simulink library "powerlib_extras"  (Simulink 6.0)
settings: Solver=ode45  SolverMode=SingleTasking  StartTime=0.0  StopTime=10.0  RelTol=1e-3
undefined symbols (not defined in the file or in its folder): Ac, Bc, Cc, Dc, Delay_discrete, dend, DiscIntNeverNeededParam, extra_sc, j, numd, test_alpha, Ts
libraries: powerlib2 x112, powerlib_extras x70, simulink_extras x25, simulink x12, powerlib_models x8
(part 3 of 9)

== system powerlib_extras/Measurements ==
  note: ____ Single-Phase Measurements _____________________________
  note: ____ Three-Phase Measurements _____________________________
  note: ____ Power Measurements __________________________________
  3-Phase Sequence Analyzer : Subsystem  mask(3-Phase Sequence analyzer){f1=60, n=1, seq=Positive}
      mask prompts: f1 "Fundamental frequency f1 (Hz):"; n "Harmonic n (0=DC; 1=fundamental) :"; seq "Sequence :"
      mask help:
      | This block outputs the positive-,  negative- or zero- or all sequence component(s) (Magnitude and Phase)  of a set of three balanced or unbalanced signals  which may contain harmonics. The three sequence components arecomputed as folllows:
      |
      | V1 = 1/3 * (Va + a*Vb  + a^2 *Vc )
      | V2 = 1/3 * (Va + a ^2*Vb  +  a *Vc )
      | V0 = 1/3 * (Va +  Vb  +  Vc )
      | where: Va, Vb, Vc = input phasors at specified frequency
      |            a =exp(j *2pi/3) = 1 < + 120 deg.  complex operator
      |
      | The input contains the vectorized signal of the three [Va Vb Vc] sinusoidal signals
      | Output one and two give respectively the magnitude (peak value) and phase (degrees) of the specified sequence component (s).
      |
      | You can modify any parameter during the simulation in order to obtain the different sequence and  harmonic components of the input. signals.
      |
      | Press Help for more information.
      mask init:
      | Pha20_On=0;
      | k=2-(n==0);
      | a=exp(j*2*pi/3);
      | a2=exp(-j*2*pi/3);
      | switch seq
      | case 1,  % Pos. seq.
      |      PosOn=1;NegOn=0;ZeroOn=0;SelectElement=1;
      | case 2,  % Neg. seq.
      |      PosOn=0;NegOn=1;ZeroOn=0;SelectElement=2;
      | case 3,  % Zero. seq.
      |      PosOn=0;NegOn=0;ZeroOn=1;SelectElement=3;
      | case 4,  % All sequences
      |      PosOn=1;NegOn=1;ZeroOn=1;SelectElement=[1,2,3];Pha20_On=1;
      | end
      mask Help: web(psbhelp)
      mask StyleString: edit,edit,popup(Positive|Negative|Zero|Positive Negative Zero)
  3-phase  Instantaneous  Active & Reactive Power : Subsystem  mask(3-phase instantaneous active and reactive power){}
      mask help:
      | This block computes the 3-phase instantaneous active (P) and reactive (Q) power associated with a periodic set of 3-phase voltages and currents.
      | Note: Result for the instantaneous reactive power (Q) is accurate only for balanced and harmonic-free 3-phase quantities (voltages and currents).
      |
      | Input 1: Vectorized 3-phase  instantaneous voltage (Vabc)
      | Input 2: Vectorized 3-phase instantaneous current (Iabc)
      | Output : Computed PQ vector [P(W) Q(var)]. Current flowing into an RL circuit will produce  positive active and reactive power.
  Active & Reactive Power : Subsystem  mask(Active & Reactive Power ){f1=60}
      mask prompts: f1 "Fundamental frequency (Hz):"
      mask help:
      | This block measures the active power P and reactive power Q  associated with a periodic  set of voltage and current which may contain harmonics. P and Q are calculated by averaging the V.I product with a running window over one cycle of the fundamental frequency so that the powers are evaluated at fundamental frequency.
      |
      | Sign convention: Current flowing into an RL branch will produce positive active and reactive powers.
      mask Help: web(psbhelp)
  Fourier : Subsystem  mask(Fourier analyser){f1=60, n=1}
      mask prompts: f1 "Fundamental frequency f1 (Hz):"; n "Harmonic n (0=DC; 1=fundamental; 2=2nd harm;  ...) :"
      mask help: The Fourier block performs a Fourier analysis of the input signal over a running window of one cycle of the fundamental frequency. First and second outputs return respectively the magnitude and phase (degrees) of the harmonic component specified.
      mask init:
      | k=2-(n==0);
      mask Help: web(psbhelp)
  Mean Value : Subsystem  mask(Mean value){Period=1/60}
      mask prompts: Period "Averaging period (s):"
      mask help: This block uses the running window averaging technique to compute the mean value of the input signal over the specified period.
  Mean Value (linear) : Subsystem  mask(Mean Value (linear)){Freq=60, n=3, Vinit=1}
      mask prompts: Freq "Fundamental frequency (Hz)"; n "Pade order (for linearization)"; Vinit "Initial input:"
      mask help:
      | This block computes the mean value of the input signal over one cycle of the specified fundamental frequency.
      | Pade approximation is used to linearize the one-cycle delay required to compute the mean value.
      mask init:
      | % Pade Approximation:
      | % The coefficients of the Pade approximation are given by the 
      | % recursion   h[k+1] = (N-k)/(2*N-k)/(k+1) * h[k],  h[0] = 1
      | % and 
      | %     exp(-T*s) == Sum { h[k] (-T*s)^k } / Sum { h[k] (T*s)^k }
      | %
      | T=1/Freq;
      | a = zeros(1,n+1);   a(1) = 1;
      | b = zeros(1,n+1);   b(1) = 1;
      | for k = 1:n,
      | 	fact = T*(n-k+1)/(2*n-k+1)/k;
      | 	a(k+1) = (-fact) * a(k);
      | 	b(k+1) = fact * b(k);
      | end
      | a = fliplr(a/b(n+1));
      | b = fliplr(b/b(n+1));
      | %
      | %Initial conditions:
      | [Ac,Bc,Cc,Dc]=tf2ss(a,b);
      | u=Vinit*exp(j*90*pi/180);
      | u0=imag(u); % input at  t=0;
      | I=eye(size(Ac));
      | x=inv(-Ac)*Bc*u;
      | x0c=imag(x);
  RMS : Subsystem  mask(RMS){f1=60}
      mask prompts: f1 "Fundamental frequency (Hz):"
      mask help: This block measures the root mean square value of instantaneous current or voltage signal connected to the input of the block. The RMS value is calculated over a running window of one cycle of the specified fundamental frequency.
      mask Help: web(psbhelp)
  Total Harmonic Distorsion : Subsystem  mask(Total Harmonic Distortion){f1=60}
      mask prompts: f1 "Fundamental frequency (Hz):"
      mask help:
      | This block measures the total harmonic distortion  (THD ) of a periodic instantaneous voltage or current connected to the input.
      | The THD is defined as:
      |
      |                   THD = Uh/U1
      | where:
      |    Uh = rms value of the harmonics
      |          = sqrt(U2^2 + U3^2 + ....+ Un^2 +...)
      |    U1 = rms value of the fundamental component
      mask Help: web(psbhelp)
  abc_to_dq0 Transformation : Subsystem
      mask Type: abc to dq0 Transformation
      mask Description:
      | This block performs the  abc to dq0 transformation on a set of three-phase signals. It computes the direct axis Vd, quadratic axis Vq, and zero sequence V0 quantities in a two axis rotating reference frame according to the following transformation:
      | 
      | Vd = 2/3*[Va*sin(wt)  + Vb*sin(wt-2pi/3)  +  Vc*sin(wt+2pi/3)]
      | Vq = 2/3*[Va*cos(wt) + Vb*cos(wt-2pi/3) + Vc*cos(wt+2pi/3)]
      | V0 = 1/3*[Va +  Vb  +  Vc ]
      | 
      | where w=  rotation speed (rad/s) of the rotating frame.
      | 
      | This transformation is commonly used in three-phase electric machine models where it is known as the Park transformation.
      mask Help: web(psbhelp);
  dq0-based Active & Reactive Power : Subsystem  AncestorBlock=|  mask(dq0-based active and reactive power computation){}
      | powerlib_extras/Discrete
      | Measurements/dq0-based
      | Active and Reactive
      | Power Computation
      mask help:
      | This block computes the instantaneous active power (P) and reactive power (Q) using as inputs 3-phase voltage and current expressed in dq0 components.
      |
      | Vectorized Input 1: direct axis, quadrature axis and zero-sequence components of the 3-phase voltage (Vdq0)
      | Vectorized Input 2: direct axis, quadrature axis and zero-sequence components of the 3-phase current (Idq0)
      |
      | Output : Computed PQ vector [P(W) Q(var)]. Current flowing into an RL circuit will produce  positive active and reactive power.
      |
      | Note: Result for the instantaneous reactive power (Q) is accurate only for balanced and harmonic-free 3-phase voltages and currents.
  dq0_to_abc Transformation : Subsystem
      mask Type: dq0 to abc Transformation
      mask Description:
      | This block transforms  three quantities  (direct axis, quadature axis and zero-sequence components)  expressed in a two axis reference frame back to phase quantities.
      | 
      | The following transformation is used:
      | 
      | Va = [Vd*sin(wt) +  Vq*cos(wt)  +  Vo ]
      | Vb = [Vd*sin(wt-2pi/3)  + Vq*cos(wt-2pi/3)  + Vo)
      | Vc = [Vd*sin(wt+2pi/3) + Vq*cos(wt+2pi/3)  + Vo)
      | where w=  rotation speed (rad/s) of the rotating frame.
      | 
      | Input 1 contains  the vectorized signal of [Vd Vq  Vo] components
      | Input 2 must contain a  [sin(wt)  cos(wt)] two dimension signal , where w is the rotation speed  of the reference frame.
      | Output is a vectozized signal containing the three  [Va Vb Vc] phase sinusoidal quantities.
      | 
      | Press Help for more information.
      mask Help: web(psbhelp)

== system powerlib_extras/Phasor Library ==
  note: ____ FACTS ___________________________
  note: ____ Measurements ____________________
  note: (Version 2.3 only)
  3-Phase Active & Reactive Power (Phasor Type) : Subsystem
      mask Type: 3-Phase Active & Reactive Power (Phasor Type)
      mask Description: 3-Phase Active & Reactive Power (Phasor Type)
  Active & Reactive Power (Phasor Type) : Subsystem
      mask Type: Active & Reactive Power (Phasor Type)
      mask Description: Active & Reactive Power (Phasor Type)
  Mean Value (Phasor Type) : Subsystem  mask(Mean value (phasor type)){Period=1/60}
      mask prompts: Period "Averaging period (s):"
      mask help: This block uses the running window averaging technique to compute the mean value of the input phasor over the specified period.
  Sequence Analyzer (Phasor Type) : Subsystem  mask(Sequence Analyzer (Phasor Type)){seq=Positive}
      mask prompts: seq "Sequence:"
      mask help:
      | This block outputs the positive-,  negative- or zero- or all sequence component(s) (Magnitude and Phase)  of a set of three  phasors. The three sequence components are computed as follows:
      |
      | V1 = 1/3 * (Va + a*Vb  + a^2 *Vc )
      | V2 = 1/3 * (Va + a ^2*Vb  +  a *Vc )
      | V0 = 1/3 * (Va +  Vb  +  Vc )
      | where: Va, Vb, Vc = input phasors
      |            a =exp(j *2pi/3) = 1 < + 120 deg.  complex operator
      |
      | The input contains the vectorized signal of the three [Va Vb Vc] phasors
      | Output one and two give respectively the magnitude (peak value) and phase (degrees) of the specified sequence component (s)
      | .
      mask init:
      | a=exp(j*2*pi/3);
      | a2=exp(-j*2*pi/3);
      | %
      | switch seq
      | case 1,  % Pos. seq.
      |      PosOn=1;NegOn=0;ZeroOn=0;SelectElement=1;
      | case 2,  % Neg. seq.
      |      PosOn=0;NegOn=1;ZeroOn=0;SelectElement=2;
      | case 3,  % Zero. seq.
      |      PosOn=0;NegOn=0;ZeroOn=1;SelectElement=3;
      | case 4,  % All sequences
      | PosOn=1;
      | NegOn=1; ZeroOn=1; SelectElement=[1,2,3];
      | end
      mask StyleString: popup(Positive|Negative|Zero|Positive Negative Zero)
  Static Var Compensator (Phasor Type) : Subsystem  mask(Static Var Compensator (Phasor Type)){mode=Fixed Susceptance, Vnom=500e3, Qnom=200e6, Bref=0.0, Vref=1.009, Xs=0.03, To=0.1, Tm=8e-3, Td=4e-3}
      mask prompts: mode "Mode of operation"; Vnom "Nominal voltage (Vrms Ph-Ph):"; Qnom "Nominal reactive power (var):"; Bref "Bref  for fixed susceptance mode (pu)"; Vref "Reference voltage Vref  (pu):"; Xs "Droop Xs (pu ):"; To "Open loop time constant To (s):"; Tm "Time constant of voltage measurement system Tm (s):"; Td "Average time delay due to thyristor valves firing Td (s):"
      mask help:
      | This block implements a  phasor model of a Static Var Compensator (SVC).
      |
      | Open loop time constant of voltage regulator:  To=1/(KI*Xs)
      |     where:
      |     KI = integrator gain of voltage regulator
      |           ((pu of B) /( pu of V)/s)
      |     Xs= Droop (pu on SVC nominal power)
      |
      | Closed loop time constant: Tc=To*1/(1+Xn/Xs)
      |     where:
      |     Xn = network impedance
      |            (pu on SVC nominal power)
      mask init:
      | Vbase=Vnom/sqrt(3)*sqrt(2);
      | Ibase=Qnom/Vnom/sqrt(3)*sqrt(2);
      | Ki=1/To/Xs;
      settings: CloseFcn=%3phaseVImeasurement
      mask StyleString: popup(Automatic|Fixed Susceptance),edit,edit,edit,edit,edit,edit,edit,edit

== system powerlib_extras/Three-Phase Library ==
  3- Phase Parallel RLC : powerlib2/Elements/3-Phase Parallel RLC Branch  R=1  L=1e-3  C=1e-6
  3- Phase RLC Series Load : powerlib2/Elements/3-Phase Series RLC Load  Vpp=500e3  fn=60  P3=50e6  QL3=25e6  QC3=200e6
  "3- Phase Series RLC " : powerlib2/Elements/3-Phase Series RLC Branch   R=1  L=1e-3  C=1e-6
  3-Phase Breaker : powerlib2/Elements/3-Phase Breaker  init_states=open  sa=on  sb=on  sc=on  sw_times="[4/60  10/60]"  Ts=0  comext=off  Ron=0.001  Rp=1e6  Cp=inf  mesure=None
  3-Phase Fault : powerlib2/Elements/3-Phase Fault  sa=on  sb=on  sc=on  Rdef=0.001  st=on  Rt=0.001  comext=on  sw_status=[1 0]  sw_times=[ 1/60 5/60]  Ts=0  init_statext=[0 0 1]  Rp=1e6  Cp=inf  mesure=None
  3-Phase RLC Parallel Load : powerlib2/Elements/3-Phase Parallel RLC Load  Vpp=500e3  fn=60  P3=50e6  QL3=25e6  QC3=200e6
  6 - pulse  diode  bridge : Subsystem  mask(Six-pulse diode bridge){Ron=0.01, Lon=10e-6, Vf=0.8, Rs=2000, Cs=50e-9}
      mask prompts: Ron "Diode on-state resitance (Ohms) :"; Lon "Diode on-state inductance (H) :"; Vf "Diode forward voltage (V) :"; Rs "Snubber resistance (Ohms) :"; Cs "Snubber capacitance (F) :"
      mask help: This block implements a six-pulses diode bridge rectifier with RC snubbers. Set the snubber resistance to Inf to remove all the diode snubbers. This block uses six diodes blocks from the powerlib/Power Electronics library.
      mask Display: plot(0,0,100,100,[50,50,35,50,65,50],[30,40,40,60,40,40],[35,65],[60,60],[50,50],[60,70])
  6 - pulse  thyristor bridge : Subsystem  mask(Six-pulse thyristor bridge){Ron=0.01, Lon=10e-6, Rs=2000, Cs=50e-9}
      mask prompts: Ron "Thyristor on-state resitance (Ohms) :"; Lon "Thyristor on-state inductance (H) :"; Rs "Snubber resistance (Ohms) :"; Cs "Snubber capacitance (F) :"
      mask help:
      | This block implements a six-pulses thyristor bridge rectifier with RC snubbers. Set the snubber resistance to Inf to remove all the thyristors snubbers. This block uses six Simplified Thyristors from the powerlib/Power Electronics library.
      | Input four (labeled 'pulses') of the block is a Simulink vector of length six that  controls the thyristors gates. Use the 'Look Under Mask' in the Edit menu  to see how the control vector operates the six thyrsistors.
      mask Display: plot(0,0,100,100,[50,50,35,50,65,50],[30,40,40,60,40,40],[35,65],[60,60],[50,50],[60,70],[45,40],[60,65],[35,40],[65,65])
  DYg linear transformer : Subsystem  mask(Delta / Y  linear tranformer){pf=[ 300e6 60 ], urx1=[ 13.8e3 0.0025  0.1 ], urx2=[ 315e3 0.0025 0.1], rxm=[ 500 500 ]}
      mask prompts: pf "[Three-phase rated power(VA)  Frequency (Hz)]"; urx1 "Winding 1 (Delta) : [Ph-Ph Voltage(Vrms)  R(pu)  X(pu)] :"; urx2 "Winding 2 (Yg) :    [Ph-Ph voltage(Vrms)  R(pu)  X(pu)] :"; rxm "Magnetizing branch : [Rm(pu)  Xm(pu)] :"
      mask help:
      | This block implements a three-phase linear transformer by using three single-phase linear transformers.
      | Winding one is connected in Delta configuration.
      | Winding two is connected in Y configuration with neutral connected to the ground.
      mask init:
      | pnom=pf(1)/3; fnom=pf(2);
      | u1=urx1(1); r1=urx1(2); x1=urx1(3);
      | u2=urx2(1)/sqrt(3); r2=urx2(2); x2=urx2(3);
      mask Display:
      | plot(0,0,100,100,[55,70,70],[35,50,65],[70,85],[50,35]);
      | plot(0,0,100,100,[70,70],[50,40],[63,77],[40,40],[65,75],[38,38],[67,73],[36,36])
      | plot(0,0,100,100,[20,20,35,20],[65,35,50,65])
  Inductive source with neutral : Subsystem  mask(3-phase inductive source - Ungrounded neutral){V=1000, Phi=-30, F=60, R=0.724, L=19.2e-3}
      mask prompts: V "Phase-to-ground peak voltage (V) :"; Phi "Phase angle of phase A (Degrees) :"; F "Frequency (Hz) :"; R "Source resistance (Ohms):"; L "Source inductance (H) :"
      mask help: This block implements a three-phase source in series with a serie RL branch. the common node (neutral) of the three sources is accesible via input one (N) of the block
      mask init:
      | [s1,s2,s3,s4]=powericon('3-phase inductive source - Ungrounded neutral',R,L);
      mask Help: Look under the mask of the 3-phase inductive source - Ungrounded neutral block to see how it is built.
      mask Display:
      | plot(-170,-60,360,60,s1,s2,s3,s4, [0,9,18,24,29,30,29,24,18,9,0,-9,-18,-24,-29,-30,-29,-24,-18,-9,0]*1.5-45,
      | [30,29,24,18,9,0,-9,-18,-24,-29,-30,-29,-24,-18,-9,0,9,18,24,29,30]*0.8,[-150,-90],[0,0])
  PI Line Section : powerlib2/Elements/3-Phase PI Section  f=60  R10=[ 0.01273 0.3864]  L10="[ 0.9337e-3  4.1264e-3]"  C10=[12.74e-9 7.751e-9]  long=100
  "Three-phase  Linear Transformer 12-terminals " : powerlib2/Elements/3-Phase Transformer 12-terminals  pf=[ 10e6 60 ]  urx1="[ 10e3 0.002  0.05 ]"  urx2=[ 25e3 0.002 0.05]  rxm=[ 200 200 ]
  "YgD  linear transformer " : Subsystem  mask(Y / Delta linear transformer){pf=[ 300e6 60 ], urx1=[ 13.8e3 0.0025  0.1 ], urx2=[ 315e3 0.0025 0.1], rxm=[ 500 500 ]}
      mask prompts: pf "[Three-phase rated power(VA)  Frequency (Hz)]"; urx1 "Winding 1 (Yg) :    [Ph-Ph Voltage(Vrms)  R(pu)  X(pu)] :"; urx2 "Winding 2 (Delta) :[Ph-Ph voltage(Vrms)  R(pu)  X(pu)] :"; rxm "Magnetizing branch : [Rm(pu)  Xm(pu)] :"
      mask help:
      | This block implements a three-phase linear transformer by using three single-phase linear transformers.
      | Winding one is in Y configuration with neutral connected to the ground.
      | Winding two is in Delta configuration.
      mask init:
      | pnom=pf(1)/3; fnom=pf(2);
      | u1=urx1(1)/sqrt(3); r1=urx1(2); x1=urx1(3);
      | u2=urx2(1); r2=urx2(2); x2=urx2(3);
      mask Display:
      | plot(0,0,100,100,[15,30,30],[35,50,65],[30,45],[50,35]);
      | plot(0,0,100,100,[30,30],[50,40],[23,37],[40,40],[25,35],[38,38],[27,33],[36,36])
      | plot(0,0,100,100,[60,60,75,60],[65,35,50,65])
  "YgY linear transformer " : Subsystem  mask(Y / Y linear transformer){pf=[ 1196e6 50 ], urx1=[ 345e3 0.003  0.09], urx2=[ 389.8e3 0.003 0.09], rxm=[ 500 500 ]}
      mask prompts: pf "[Three-phase rated power(VA)  Frequency (Hz)]"; urx1 "Winding 1 (Yg) : [Ph-Ph Voltage(Vrms)  R(pu)  X(pu)] :"; urx2 "Winding 2 (Y) :  [Ph-Ph voltage(Vrms)  R(pu)  X(pu)] :"; rxm "Magnetizing branch : [Rm(pu)  Xm(pu)] :"
      mask help:
      | This block implements a three-phase linear transformer by using three single-phase linear transformers.
      | Winding one is connected in Y configuration with neutral connected to the ground.
      | Winding two is connected in Y configuration with a floating neutral.
      mask init:
      | pnom=pf(1)/3; fnom=pf(2);
      | u1=urx1(1)/sqrt(3); r1=urx1(2); x1=urx1(3);
      | u2=urx2(1)/sqrt(3); r2=urx2(2); x2=urx2(3);
      mask Display:
      | plot(0,0,100,100,[15,30,30],[35,50,65],[30,45],[50,35]);
      | plot(0,0,100,100,[30,30],[50,40],[23,37],[40,40],[25,35],[38,38],[27,33],[36,36])
      | plot(0,0,100,100,[55,70,70],[35,50,65],[70,85],[50,35])
  YgYD linear transformer : Subsystem  mask(Y / Y-Delta  linear transformer){pf=[ 300e6 60 ], urx1=[ 735e3 0.0025  0.1 ], urx2=[ 315e3 0.0025 0.1], urx3=[ 25e3 0.0025 0.1 ], rxm=[ 500 500 ]}
      mask prompts: pf "[Three-phase rated power(VA)  Frequency (Hz)]"; urx1 "Winding 1 (Yg) :      [Ph-Ph Voltage(Vrms)  R(pu)  X(pu)] :"; urx2 "Winding 2 (Y) :       [Ph-Ph voltage(Vrms)  R(pu)  X(pu)] :"; urx3 "Winding 3 (Delta) : [Ph-Ph voltage(Vrms)  R(pu)   X(pu)] :"; rxm "Magnetizing branch : [Rm(pu)  Xm(pu)] :"
      mask help:
      | This block implements a three phase linear transformer by using three single-phase linear transformers.
      | Winding one is connected in Y configuration with neutral connected to the ground.
      | Winding two is connected in Y configuration with a floating neutral.
      | Winding three is connected in Delta configuration.
      mask init:
      | pnom=pf(1)/3; fnom=pf(2);
      | u1=urx1(1)/sqrt(3); r1=urx1(2); x1=urx1(3);
      | u2=urx2(1)/sqrt(3); r2=urx2(2); x2=urx2(3);
      | u3=urx3(1); r3=urx3(2); x3=urx3(3);
      mask Display:
      | plot(0,0,100,100,[15,30,30],[35,50,65],[30,45],[50,35],[55,70,70],[60,75,90],[70,85],[75,60]);
      | plot(0,0,100,100,[30,30],[50,40],[25,37],[40,40],[25,35],[38,38],[27,33],[36,36])
      | plot(0,0,100,100,[65,65,80,65],[40,10,25,40])
  YgYgD linear transformer : Subsystem  mask(Y / Y-Delta  linear transformer){pf=[ 300e6 60 ], urx1=[ 735e3 0.0025  0.1 ], urx2=[ 315e3 0.0025 0.1], urx3=[ 25e3 0.0025 0.1 ], rxm=[ 500 500 ]}
      mask prompts: pf "[Three-phase rated power(VA)  Frequency (Hz)]"; urx1 "Winding 1 (Yg) :    [Ph-Ph Voltage(Vrms)  R(pu)  X(pu)] :"; urx2 "Winding 2 (Yg) :    [Ph-Ph voltage(Vrms)  R(pu)  X(pu)] :"; urx3 "Winding 3 (Delta) : [Ph-Ph voltage(Vrms)  R(pu)   X(pu)] :"; rxm "Magnetizing branch : [Rm(pu)  Xm(pu)] :"
      mask help:
      | This block implements a three phase linear transformer by using three single-phase linear transformers.
      | Winding one is connected in Y configuration with neutral connected to the ground.
      | Winding two is connected in Y configuration with neutral connected to ground.
      | Winding three is connected in Delta configuration.
      mask init:
      | pnom=pf(1)/3; fnom=pf(2);
      | u1=urx1(1)/sqrt(3); r1=urx1(2); x1=urx1(3);
      | u2=urx2(1)/sqrt(3); r2=urx2(2); x2=urx2(3);
      | u3=urx3(1); r3=urx3(2); x3=urx3(3);
      mask Display:
      | plot(0,0,100,100,[15,30,30],[35,50,65],[30,45],[50,35],[55,70,70],[60,75,90],[70,85],[75,60]);
      | plot(0,0,100,100,[30,30],[50,40],[25,37],[40,40],[25,35],[38,38],[27,33],[36,36])
      | plot(0,0,100,100,[70,70],[75,65],[63,77],[65,65],[65,75],[63,63],[67,73],[61,61])
      | plot(0,0,100,100,[65,65,80,65],[40,10,25,40])
  YgYgD saturable transformer : Subsystem  mask(Y / Y-Delta  Saturable transformer){pf=[ 450e6 60 ], urx1=[ 500e3 0.002 0.08 ], urx2=[ 230e3 0.002 0.08], urx3=[ 60e3 0.015 0.30], sat=[0 0; 0.0 1.2; 1.0  1.52], Rm=500, phi0=[0.8 -0.4 0.4]}
      mask prompts: pf "[Three-phase rated power(VA)  Frequency (Hz)]"; urx1 "Winding 1 (Yg) :    [Ph-Ph Voltage(Vrms)  R(pu)  X(pu)] :"; urx2 "Winding 2 (Yg) :    [Ph-Ph voltage(Vrms)  R(pu)  X(pu)] :"; urx3 "Winding 3 (Delta) : [Ph-Ph voltage(Vrms)  R(pu)   X(pu)] :"; sat "Saturation characterstic [i1(pu) phi1(pu); i2 phi2; ...]"; Rm "Core loss resistance Rm (pu) :"; phi0 "Residual fluxes (pu)  [phi0A  phi0B phi0C] or 'auto'"
      mask help:
      | This block implements a three phase Saturable transformer by using three single-phase saturable transformers.
      | Winding one is connected in Y configuration with neutral connected to the ground.
      | Winding two is connected in Y configuration with neutral connected to ground.
      | Winding three is connected in Delta configuration.
      | Enter the saturation characteristic for one mono-phase saturable transformer. The saturation characteristic is the same for A,B, and C  phases.
      | For flux initialization, you  can either specify a vector of three resisual fluxes, or use automatic initialization  corresponding to steady state by entering the string 'auto'.
      mask init:
      | pnom=pf(1)/3; fnom=pf(2);
      | u1=urx1(1)/sqrt(3); r1=urx1(2); x1=urx1(3);
      | u2=urx2(1)/sqrt(3); r2=urx2(2); x2=urx2(3);
      | u3=urx3(1); r3=urx3(2); x3=urx3(3);
      | if  isstr(phi0) & strcmp(phi0,'auto')
      |    Rm_phi0_1=Rm;
      |    Rm_phi0_2=Rm;
      |    Rm_phi0_3=Rm;
      | else
      |    Rm_phi0_1=[Rm phi0(1)];
      |    Rm_phi0_2=[Rm phi0(2)];
      |    Rm_phi0_3=[Rm phi0(3)];
      | end
      mask Display:
      | plot(0,0,100,100,[15,30,30],[35,50,65],[30,45],[50,35],[55,70,70],[60,75,90],[70,85],[75,60]);
      | plot(0,0,100,100,[30,30],[50,40],[25,37],[40,40],[25,35],[38,38],[27,33],[36,36])
      | plot(0,0,100,100,[70,70],[75,65],[63,77],[65,65],[65,75],[63,63],[67,73],[61,61])
      | plot(0,0,100,100,[65,65,80,65],[40,10,25,40])
      | 
      | plot(0,0,100,100,[40, 50 ,50 ,60], [10,15,85,90])
  Z1-Z0 : powerlib2/Elements/3-Phase Mutual Inductance Z1-Z0  RL1="[ 2  50e-3]"  RL0="[4  100e-3]"

== system powerlib_extras/Additional Machines/Discrete DC_Machine ==
  F+ : Inport  Port=1  LatchInput=off
  A+ : Inport  Port=2  LatchInput=off
  TL : Inport  Port=3  LatchInput=off
  + : powerlib2/Connectors/L connector  Tag=PoWeRsYsTeMbLoCk  Orientation=down
  Coulomb (Tf) & Viscous ( Bm*w)  Friction Torques : simulink/Discontinuities/Coulomb & Viscous Friction  Orientation=left  offset=Tf  gain=Bm
  Discrete-Time Integrator : DiscreteIntegrator  InitialCondition=w0  SampleTime=Ts  ICPrevOutput=DiscIntNeverNeededParam  ICPrevScaledInput=DiscIntNeverNeededParam
  E_FCEM : powerlib2/Electrical Sources/Controlled Voltage Source  Tag=PoWeRsYsTeMbLoCk  Orientation=left  initsrc=on  srctyp=AC  iv=0  iph=0  ifreq=0  mesure=None  PSBOutputType=11
  Gain2 : Gain  Gain=1/J  SaturateOnIntegerOverflow=on
  Gain3 : Gain  Gain=Laf  SaturateOnIntegerOverflow=on
  Ia_mot : powerlib2/Measurements/Current Measurement  Tag=PoWeRsYsTeMmEaSuReMeNt  PhasorSimulation=off  OutputType=Complex  PSBOutputType=01  PSBequivalent=0
  Mux : Mux
  Product : Product  Orientation=left  SaturateOnIntegerOverflow=on  InputSameDT=on
  Product1 : Product  SaturateOnIntegerOverflow=on  InputSameDT=on
  Product2 : Product  SaturateOnIntegerOverflow=on  InputSameDT=on
  Ra  La : powerlib2/Elements/Series RLC Branch  Tag=PoWeRsYsTeMbLoCk  Orientation=down  a=Ra  b=La  c=inf  mesure=None  PSBOutputType=1
  Rf  Lf : powerlib2/Elements/Series RLC Branch  Tag=PoWeRsYsTeMbLoCk  Orientation=down  a=Rf  b=Lf  c=inf  mesure=None  PSBOutputType=1
  Sign : Signum  Orientation=left
  Sum : Sum  Inputs=-+-  SaturateOnIntegerOverflow=on  InputSameDT=on
  Unit Delay : UnitDelay  SampleTime=Ts
  if : powerlib2/Measurements/Current Measurement  Tag=PoWeRsYsTeMmEaSuReMeNt  PhasorSimulation=off  OutputType=Complex  PSBOutputType=01  PSBequivalent=0
  F- : Outport  Orientation=left  InitialOutput=0
  A- : Outport  Orientation=left  Port=2  InitialOutput=0
  m : Outport  Port=3  InitialOutput=0
  wires:
  Coulomb (Tf) & Viscous ( Bm*w)  Friction Torques/1 -> Sum/3
  Mux/1 -> m/1
  Product1/1 -> Mux/4, Sum/2  "Te"
  Product/1 -> E_FCEM/1
  Discrete-Time Integrator/1 -> Sign/1, Mux/1, Product/1, Coulomb (Tf) & Viscous ( Bm*w)  Friction Torques/1  "w"
  Gain2/1 -> Discrete-Time Integrator/1
  Sum/1 -> Gain2/1
  Sign/1 -> Product2/1
  TL/1 -> Product2/2
  Product2/1 -> Sum/1
  if/1 -> Mux/3, Gain3/1  "If"
  Ia_mot/1 -> Mux/2, Product1/1  "Ia"
  Rf  Lf/1 -> F-/1
  E_FCEM/2 -> A-/1
  E_FCEM/1 -> +/Enable
  if/2 -> Rf  Lf/1
  F+/1 -> if/1
  Ra  La/1 -> +/1
  Ia_mot/2 -> Ra  La/1
  A+/1 -> Ia_mot/1
  Gain3/1 -> Unit Delay/1
  Unit Delay/1 -> Product/2, Product1/2

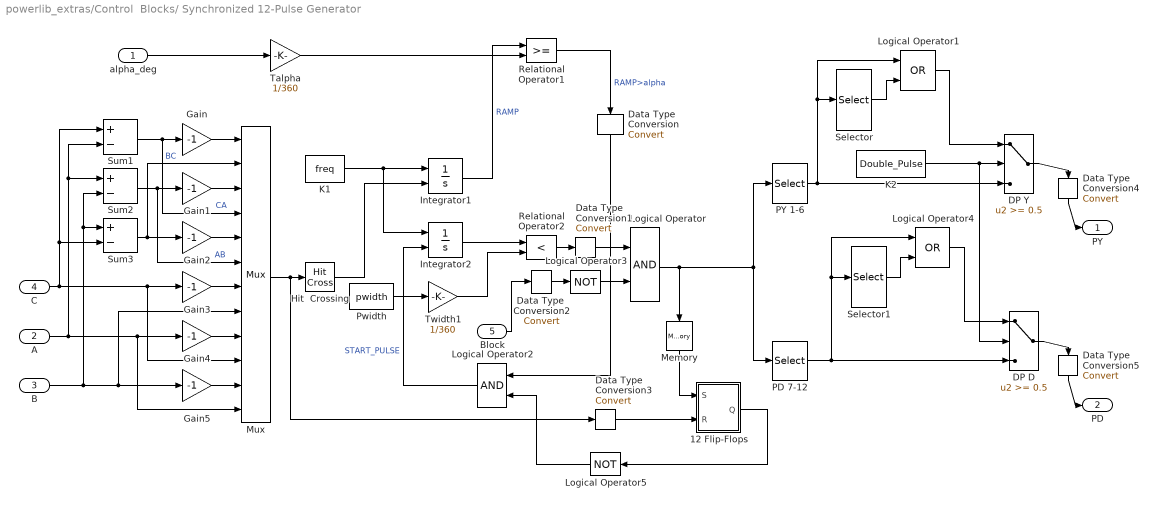
== system powerlib_extras/Control  Blocks/ Synchronized 12-Pulse Generator ==
  alpha_deg : Inport  Port=1  LatchInput=off
  A : Inport  Port=2  LatchInput=off
  B : Inport  Port=3  LatchInput=off
  C : Inport  Port=4  LatchInput=off
  Block : Inport  Port=5  LatchInput=off
  12 Flip-Flops : Subsystem
  DP D : Switch  Threshold=0.5  InputSameDT=on
  DP Y : Switch  Threshold=0.5  InputSameDT=on
  Data Type  Conversion : DataTypeConversion  Orientation=down  OutDataTypeMode=boolean  SaturateOnIntegerOverflow=on  RndMeth=Zero
  Data Type  Conversion1 : DataTypeConversion  OutDataTypeMode=boolean  SaturateOnIntegerOverflow=on  RndMeth=Zero
  Data Type  Conversion2 : DataTypeConversion  OutDataTypeMode=boolean  SaturateOnIntegerOverflow=on  RndMeth=Zero
  Data Type  Conversion3 : DataTypeConversion  OutDataTypeMode=boolean  SaturateOnIntegerOverflow=on  RndMeth=Zero
  Data Type  Conversion4 : DataTypeConversion  Orientation=down  OutDataTypeMode=double  SaturateOnIntegerOverflow=on  RndMeth=Zero
  Data Type  Conversion5 : DataTypeConversion  Orientation=down  OutDataTypeMode=double  SaturateOnIntegerOverflow=on  RndMeth=Zero
  Gain{,1..5} (6 alike) : Gain  Gain=-1  SaturateOnIntegerOverflow=on
  Hit  Crossing : HitCross  HitCrossingDirection=rising
  Integrator1 : Integrator  ExternalReset=rising
  Integrator2 : Integrator  ExternalReset=rising
  K1 : Constant  Value=freq
  K2 : Constant  Value=Double_Pulse
  Logical Operator : Logic
  Logical Operator1 : Logic  Operator=OR
  Logical Operator2 : Logic  Orientation=left
  Logical Operator3 : Logic  Operator=NOT  Inputs=1
  Logical Operator4 : Logic  Operator=OR
  Logical Operator5 : Logic  Orientation=left  Operator=NOT  Inputs=1
  Memory : Memory  Orientation=down
  Mux : Mux  Inputs=12
  PD 7-12 : Selector  Elements=7:12  InputPortWidth=12
  PY 1-6 : Selector  Elements=1:6  InputPortWidth=12
  Pwidth : Constant  Value=pwidth
  Relational Operator1 : RelationalOperator  InputSameDT=on
  Relational Operator2 : RelationalOperator  Operator=<  InputSameDT=on
  Selector : Selector  Elements=[2 3 4 5 6 1 ]  InputPortWidth=6
  Selector1 : Selector  Elements=[2 3 4 5 6 1 ]  InputPortWidth=6
  Sum1 : Sum  Inputs=+-  SaturateOnIntegerOverflow=on  InputSameDT=on
  Sum2 : Sum  Inputs=+-  SaturateOnIntegerOverflow=on  InputSameDT=on
  Sum3 : Sum  Inputs=+-  SaturateOnIntegerOverflow=on  InputSameDT=on
  Talpha : Gain  Gain=1/360  SaturateOnIntegerOverflow=on
  Twidth1 : Gain  Gain=1/360  SaturateOnIntegerOverflow=on
  PY : Outport  InitialOutput=0
  PD : Outport  Port=2  InitialOutput=0
  wires:
  Mux/1 -> Hit  Crossing/1
  Gain2/1 -> Mux/5
  Gain1/1 -> Mux/3
  Gain/1 -> Mux/1
  alpha_deg/1 -> Talpha/1
  Sum1/1 -> Gain/1, Mux/4  "CA"
  Sum2/1 -> Gain1/1, Mux/6  "AB"
  Sum3/1 -> Gain2/1, Mux/2  "BC"
  Gain3/1 -> Mux/7
  Gain4/1 -> Mux/9
  Gain5/1 -> Mux/11
  C/1 -> Gain3/1, Mux/10, Sum1/1, Sum3/2
  A/1 -> Gain4/1, Mux/12, Sum2/1, Sum1/2
  B/1 -> Gain5/1, Mux/8, Sum3/1, Sum2/2
  Integrator1/1 -> Relational Operator1/1  "RAMP"
  Talpha/1 -> Relational Operator1/2
  Integrator2/1 -> Relational Operator2/1
  Twidth1/1 -> Relational Operator2/2
  Logical Operator2/1 -> Integrator2/2  "START_PULSE"
  Logical Operator5/1 -> Logical Operator2/2
  Hit  Crossing/1 -> Integrator1/2, Data Type  Conversion3/1
  Pwidth/1 -> Twidth1/1
  K1/1 -> Integrator2/1, Integrator1/1
  Memory/1 -> 12 Flip-Flops/1(S)
  Logical Operator3/1 -> Logical Operator/2
  12 Flip-Flops/1(Q) -> Logical Operator5/1
  Logical Operator/1 -> Memory/1, PY 1-6/1, PD 7-12/1
  Logical Operator1/1 -> DP Y/1
  Selector/1 -> Logical Operator1/2
  PY 1-6/1 -> DP Y/3, Selector/1, Logical Operator1/1
  Logical Operator4/1 -> DP D/1
  Selector1/1 -> Logical Operator4/2
  PD 7-12/1 -> Logical Operator4/1, Selector1/1, DP D/3
  K2/1 -> DP Y/2, DP D/2
  Relational Operator1/1 -> Data Type  Conversion/1  "RAMP>alpha"
  Data Type  Conversion/1 -> Logical Operator2/1
  Relational Operator2/1 -> Data Type  Conversion1/1
  Data Type  Conversion1/1 -> Logical Operator/1
  Block/1 -> Data Type  Conversion2/1
  Data Type  Conversion2/1 -> Logical Operator3/1
  Data Type  Conversion3/1 -> 12 Flip-Flops/2(R)
  DP Y/1 -> Data Type  Conversion4/1
  Data Type  Conversion4/1 -> PY/1
  DP D/1 -> Data Type  Conversion5/1
  Data Type  Conversion5/1 -> PD/1

== system powerlib_extras/Control  Blocks/1-phase  PLL ==
  note: 1-phase PLL
  note: Pierre Giroux, Gilbert Sybille
      | Power System Laboratory, IREQ
      | Hydro-Quebec
  note: Note: sin( a ) * cos( b )= 1/2 * sin( a+b ) + 1/2 * sin(a-b)
  V (pu) : Inport  Port=1  PortDimensions=1  LatchInput=off
  2nd-Order Filter : powerlib_extras/Control  Blocks/2nd-Order Filter  FilterType=Lowpass  Fo=25  Zeta=0.707  Initialize=on  Vac_Init=[0 0 60]  Vdc_Init=Finit  PlotResponse=off  param1=[1 1000 0.5]
  Constant4 : Constant  Value=2*pi
  Discrete PI Controller : Subsystem  mask(PI Controller){Kp=Kp, Ki=Ki, Par_Limits=2*pi*Finit*[1.25 0.75], Init=2*pi*Finit}
      mask prompts: Kp "Proportional gain (Kp):"; Ki "Integral gain (Ki):"; Par_Limits "Output limits: [ Upper   Lower ]"; Init "Output initial value:"
      mask help: This block implements a discrete PI controller.
      mask init:
      | UpperLimit=Par_Limits(1);
      | LowerLimit=Par_Limits(2);
      mask Display: disp('PI');
  Gain10 : Gain  Gain=1/2/pi  SaturateOnIntegerOverflow=on
  Integrator : Integrator  InitialCondition=Phase_Init*pi/180  LimitOutput=on
  Math Function : Math  Operator=mod  SaturateOnIntegerOverflow=on
  Mux2 : Mux  Inputs=2
  Product1 : Product  SaturateOnIntegerOverflow=on  InputSameDT=on
  Rate Limiter : RateLimiter  RisingSlewLimit=12  FallingSlewLimit=-12
  Trigonometric Function : Trigonometry
  Trigonometric Function2 : Trigonometry  Operator=cos
  Variable Frequency Mean value : Subsystem  mask(Variable-Frequency Mean Value){Finit=Finit, Vinit=0}
      mask prompts: Finit "Initial frequency (Hz):"; Vinit "Initial input (DC component):"
      mask help:
      | This  block computes the mean value of the input signal (port In) over a running window of one cycle of a specified frequency (port Freq).
      |
      | For the first cycle of simulation (specified by the parameter "Initial frequency"), the ouput is held to the value of the  "Initial input" parameter.
  Freq : Outport
  wt : Outport  Port=2
  Sin_Cos : Outport  Port=3
  wires:
  V (pu)/1 -> Product1/1
  2nd-Order Filter/1 -> Freq/1, Variable Frequency Mean value/1(Freq)
  Variable Frequency Mean value/1(Mean) -> Discrete PI Controller/1(Error)
  Constant4/1 -> Math Function/2
  Integrator/1 -> Math Function/1
  Math Function/1 -> Trigonometric Function/1, Trigonometric Function2/1, wt/1
  Trigonometric Function/1 -> Mux2/1
  Trigonometric Function2/1 -> Product1/2, Mux2/2
  Mux2/1 -> Sin_Cos/1
  Discrete PI Controller/1(Out) -> Integrator/1, Gain10/1  "W"
  Gain10/1 -> Rate Limiter/1
  Rate Limiter/1 -> 2nd-Order Filter/1
  Product1/1 -> Variable Frequency Mean value/2(In)  "Vq"

== system powerlib_extras/Control  Blocks/1st-Order  Filter ==
  In : Inport  Port=1  LatchInput=off
  State-Space : StateSpace  A=Ac  B=Bc  C=Cc  D=Dc  X0=x0c
  Out : Outport  InitialOutput=0
  wires:
  State-Space/1 -> Out/1
  In/1 -> State-Space/1

== system powerlib_extras/Control  Blocks/2nd-Order Filter ==
  In : Inport  Port=1  LatchInput=off
  State-Space : StateSpace  A=Ac  B=Bc  C=Cc  D=Dc  X0=x0c
  Out : Outport  InitialOutput=0
  wires:
  In/1 -> State-Space/1
  State-Space/1 -> Out/1

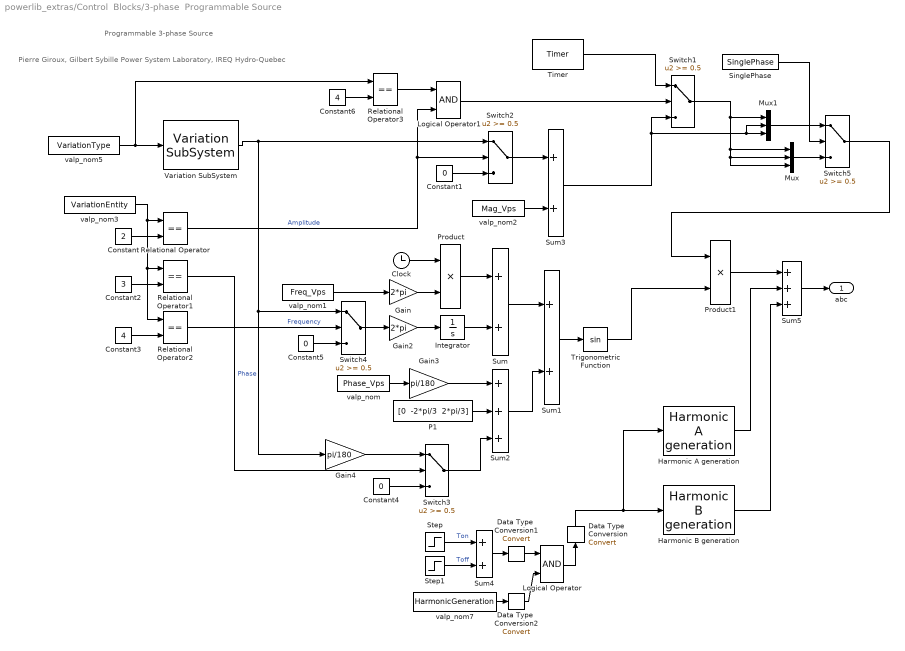
== system powerlib_extras/Control  Blocks/3-phase  Programmable Source ==
  note: Programmable 3-phase Source
  note: Pierre Giroux, Gilbert Sybille
      | Power System Laboratory, IREQ
      | Hydro-Quebec
  Clock : Clock
  Constant : Constant  Value=2
  Constant1 : Constant  Value=0
  Constant2 : Constant  Value=3
  Constant3 : Constant  Value=4
  Constant4 : Constant  Value=0
  Constant5 : Constant  Value=0
  Constant6 : Constant  Value=4
  Data Type  Conversion : DataTypeConversion  Orientation=up  OutDataTypeMode=double  SaturateOnIntegerOverflow=on  RndMeth=Zero
  Data Type  Conversion1 : DataTypeConversion  OutDataTypeMode=boolean  SaturateOnIntegerOverflow=on  RndMeth=Zero
  Data Type  Conversion2 : DataTypeConversion  OutDataTypeMode=boolean  SaturateOnIntegerOverflow=on  RndMeth=Zero
  Gain : Gain  Gain=2*pi  SaturateOnIntegerOverflow=on
  Gain2 : Gain  Gain=2*pi  SaturateOnIntegerOverflow=on
  Gain3 : Gain  Gain=pi/180  SaturateOnIntegerOverflow=on
  Gain4 : Gain  Gain=pi/180  SaturateOnIntegerOverflow=on
  Harmonic A generation : powerlib_models/Continuous/3_Phase_Prog_Source/Harmonic A generation  Freq_Vps=Freq_Vps  n_Harmo=n_HarmoA  Mag_Harmo=Mag_HarmoA  Phase_Harmo=Phase_HarmoA  Seq_Harmo=Seq_HarmoA  Ts=0
  Harmonic B generation : powerlib_models/Continuous/3_Phase_Prog_Source/Harmonic B generation  Freq_Vps=Freq_Vps  n_Harmo=n_HarmoB  Mag_Harmo=Mag_HarmoB  Phase_Harmo=Phase_HarmoB  Seq_Harmo=Seq_HarmoB  Ts=0
  Integrator : Integrator
  Logical Operator : Logic
  Logical Operator1 : Logic
  Mux : Mux  Inputs=3
  Mux1 : Mux  Inputs=3
  P1 : Constant  Value="[0  -2*pi/3  2*pi/3]"
  Product : Product  SaturateOnIntegerOverflow=on  InputSameDT=on
  Product1 : Product  SaturateOnIntegerOverflow=on  InputSameDT=on
  Relational Operator{,1..3} (4 alike) : RelationalOperator  Operator===  InputSameDT=on
  SinglePhase : Constant  Value=SinglePhase
  Step : Step  Time=Ton_Harmo  SampleTime=0
  Step1 : Step  Time=Toff_Harmo  After=-1  SampleTime=0
  Sum{,1,3..4} (4 alike) : Sum  SaturateOnIntegerOverflow=on  InputSameDT=on
  Sum2 : Sum  Inputs=+++  SaturateOnIntegerOverflow=on  InputSameDT=on
  Sum5 : Sum  Inputs=+++  SaturateOnIntegerOverflow=on  InputSameDT=on
  Switch{1..5} (5 alike) : Switch  Threshold=0.5  InputSameDT=on
  Timer : powerlib_models/Continuous/3_Phase_Prog_Source/Timer  t=Xtime  e=Yampli  Ts=0
  Trigonometric Function : Trigonometry
  Variation SubSystem : powerlib_models/Continuous/3_Phase_Prog_Source/Variation SubSystem  VariationStep=VariationStep  VariationRate=VariationRate  VariationFreq=VariationFreq  VariationMag=VariationMag  Ton_Variation=Ton_Variation  Toff_Variation=Toff_Variation  Ts=0
  valp_nom : Constant  Value=Phase_Vps
  valp_nom1 : Constant  Value=Freq_Vps
  valp_nom2 : Constant  Value=Mag_Vps
  valp_nom3 : Constant  Value=VariationEntity
  valp_nom5 : Constant  Value=VariationType
  valp_nom7 : Constant  Value=HarmonicGeneration
  abc : Outport  InitialOutput=0
  wires:
  Data Type  Conversion2/1 -> Logical Operator/2
  valp_nom7/1 -> Data Type  Conversion2/1
  Data Type  Conversion1/1 -> Logical Operator/1
  Sum4/1 -> Data Type  Conversion1/1
  Data Type  Conversion/1 -> Harmonic B generation/1, Harmonic A generation/1
  Logical Operator/1 -> Data Type  Conversion/1
  Product/1 -> Sum/1
  Gain/1 -> Product/2
  Clock/1 -> Product/1
  Sum/1 -> Sum1/1
  Sum1/1 -> Trigonometric Function/1
  Gain2/1 -> Integrator/1
  Integrator/1 -> Sum/2
  P1/1 -> Sum2/2
  Trigonometric Function/1 -> Product1/2
  Gain3/1 -> Sum2/1
  valp_nom/1 -> Gain3/1
  valp_nom1/1 -> Gain/1
  Product1/1 -> Sum5/1
  Switch2/1 -> Sum3/1
  Constant1/1 -> Switch2/3
  Sum2/1 -> Sum1/2
  valp_nom2/1 -> Sum3/2
  Relational Operator/1 -> Switch2/2, Logical Operator1/2  "Amplitude"
  valp_nom5/1 -> Variation SubSystem/1, Relational Operator3/1
  Switch3/1 -> Sum2/3
  Constant4/1 -> Switch3/3
  Relational Operator1/1 -> Switch3/2  "Phase"
  Variation SubSystem/1 -> Switch2/1, Switch4/1, Gain4/1
  Switch4/1 -> Gain2/1
  Relational Operator2/1 -> Switch4/2  "Frequency"
  Constant/1 -> Relational Operator/2
  valp_nom3/1 -> Relational Operator/1, Relational Operator2/1, Relational Operator1/1
  Constant2/1 -> Relational Operator1/2
  Constant3/1 -> Relational Operator2/2
  Constant5/1 -> Switch4/3
  Harmonic A generation/1 -> Sum5/2
  Sum5/1 -> abc/1
  Step/1 -> Sum4/1  "Ton"
  Step1/1 -> Sum4/2  "Toff"
  Harmonic B generation/1 -> Sum5/3
  Gain4/1 -> Switch3/1
  Constant6/1 -> Relational Operator3/2
  Sum3/1 -> Switch1/3, Mux1/3, Mux1/2
  Timer/1 -> Switch1/1
  Mux1/1 -> Switch5/1
  SinglePhase/1 -> Switch5/2
  Mux/1 -> Switch5/3
  Switch1/1 -> Mux/1, Mux/2, Mux/3, Mux1/1
  Switch5/1 -> Product1/1
  Relational Operator3/1 -> Logical Operator1/1
  Logical Operator1/1 -> Switch1/2

== system powerlib_extras/Control  Blocks/3-phase PLL ==
  note: 3-phase PLL
  note: Pierre Giroux, Gilbert Sybille
      | Power System Laboratory, IREQ
      | Hydro-Quebec
  Vabc (pu) : Inport  Port=1  PortDimensions=3  LatchInput=off
  2nd-Order Filter : powerlib_extras/Control  Blocks/2nd-Order Filter  FilterType=Lowpass  Fo=25  Zeta=0.707  Initialize=on  Vac_Init=[0 0 60]  Vdc_Init=Finit  PlotResponse=off  param1=[1 1000 0.5]
  Constant4 : Constant  Value=2*pi
  Discrete PI Controller : Subsystem  mask(Discrete PI Controller){Kp=Kp, Ki=Ki, Par_Limits=2*pi*Finit*[1.25 0.75], Init=2*pi*Finit}
      mask prompts: Kp "Proportional gain (Kp):"; Ki "Integral gain (Ki):"; Par_Limits "Output limits: [ Upper   Lower ]"; Init "Output initial value:"
      mask help: This block implements a discrete PI controller.
      mask init:
      | UpperLimit=Par_Limits(1);
      | LowerLimit=Par_Limits(2);
      mask Display: disp('PI');
  Gain10 : Gain  Gain=1/2/pi  SaturateOnIntegerOverflow=on
  Integrator : Integrator  InitialCondition=Phase_Init*pi/180  LimitOutput=on
  Math Function : Math  Operator=mod  SaturateOnIntegerOverflow=on
  Mux2 : Mux  Inputs=2
  Rate Limiter : RateLimiter  RisingSlewLimit=12  FallingSlewLimit=-12
  Selector : Selector  Elements=2  InputPortWidth=3
  Trigonometric Function : Trigonometry
  Trigonometric Function2 : Trigonometry  Operator=cos
  Variable Frequency Mean value : Subsystem  mask(Variable-Frequency Mean Value){Finit=Finit, Vinit=0}
      mask prompts: Finit "Initial frequency (Hz):"; Vinit "Initial input (DC component):"
      mask help:
      | This  block computes the mean value of the input signal (port In) over a running window of one cycle of a specified frequency (port Freq).
      |
      | For the first cycle of simulation (specified by the parameter "Initial frequency"), the ouput is held to the value of the  "Initial input" parameter.
  abc_to_dq0 Transformation : powerlib_extras/Measurements/abc_to_dq0 Transformation
  Freq : Outport
  wt : Outport  Port=2
  Sin_Cos : Outport  Port=3
  wires:
  2nd-Order Filter/1 -> Freq/1, Variable Frequency Mean value/1(Freq)
  Variable Frequency Mean value/1(Mean) -> Discrete PI Controller/1(Error)
  Vabc (pu)/1 -> abc_to_dq0 Transformation/1
  abc_to_dq0 Transformation/1 -> Selector/1
  Constant4/1 -> Math Function/2
  Integrator/1 -> Math Function/1
  Math Function/1 -> Trigonometric Function/1, Trigonometric Function2/1, wt/1
  Trigonometric Function/1 -> Mux2/1
  Trigonometric Function2/1 -> Mux2/2
  Mux2/1 -> abc_to_dq0 Transformation/2, Sin_Cos/1
  Discrete PI Controller/1(Out) -> Integrator/1, Gain10/1  "W"
  Gain10/1 -> Rate Limiter/1
  Rate Limiter/1 -> 2nd-Order Filter/1
  Selector/1 -> Variable Frequency Mean value/2(In)  "Vq"

== system powerlib_extras/Control  Blocks/Bistable ==
  note: Silvano Casoria
      | Power System Simulation Laboratory
      | IREQ, Hydro-Quebc
  note: Discrete Bistable Flip-Flop with priority to Set or Reset
  S : Inport  Port=1  LatchInput=off
  R : Inport  Port=2  LatchInput=off
  Constant : Constant
  Constant2 : Constant  Value=priority
  Data Type Conversion1 : DataTypeConversion  OutDataTypeMode=boolean  SaturateOnIntegerOverflow=on  RndMeth=Zero
  Data Type Conversion2 : DataTypeConversion  OutDataTypeMode=boolean  SaturateOnIntegerOverflow=on  RndMeth=Zero
  Logical Operator1 : Logic  Operator=OR
  Logical Operator2 : Logic  Operator=NOT  Inputs=1
  Logical Operator3 : Logic  Operator=OR
  RESET Priority : Subsystem  TreatAsAtomicUnit=on
  Relational Operator1 : RelationalOperator  Operator=>  InputSameDT=on
  SET  Priority : Subsystem  TreatAsAtomicUnit=on
  Q : Outport  InitialOutput=0
  !Q : Outport  Port=2  InitialOutput=1
  wires:
  RESET Priority/2(!Q) -> Logical Operator3/2
  RESET Priority/1(Q) -> Logical Operator1/2
  Logical Operator3/1 -> !Q/1
  SET  Priority/2(!Q) -> Logical Operator3/1
  Logical Operator1/1 -> Q/1
  SET  Priority/1(Q) -> Logical Operator1/1
  Constant/1 -> Relational Operator1/2
  Relational Operator1/1 -> SET  Priority/Enable, Logical Operator2/1
  Constant2/1 -> Relational Operator1/1
  Logical Operator2/1 -> RESET Priority/Enable
  Data Type Conversion1/1 -> RESET Priority/2(R), SET  Priority/2(R)
  Data Type Conversion2/1 -> RESET Priority/1(S), SET  Priority/1(S)
  S/1 -> Data Type Conversion2/1
  R/1 -> Data Type Conversion1/1

== system powerlib_extras/Control  Blocks/Edge Detector ==
  note: Edge or Slope Detector
  note: Silvano Casoria
      | Power System Simulation Laboratory
      | IREQ, Hydro-Quebc
  In : Inport  Port=1  LatchInput=off
  Constant1 : Constant  Value=model
  Demux : Demux  Outputs=2
  Logical Operator1 : Logic  Operator=OR
  Memory : Memory  X0=ic  InheritSampleTime=on
  Multiport Switch : MultiPortSwitch  Inputs=3  SaturateOnIntegerOverflow=on
  NEGATIVE Edge : Subsystem  AncestorBlock=extra_sc/Edge/POSITIVE Edge  TreatAsAtomicUnit=on
  POSITIVE Edge : Subsystem  AncestorBlock=extra_sc/Delay_discrete/OFF Delay  TreatAsAtomicUnit=on
  either edge : Constant  Value=[1 1]
  neg. edge : Constant  Value=[0 1]
  pos. edge : Constant  Value=[1 0]
  Out : Outport
  wires:
  either edge/1 -> Multiport Switch/4
  Demux/2 -> NEGATIVE Edge/Enable
  Demux/1 -> POSITIVE Edge/Enable
  Multiport Switch/1 -> Demux/1
  Constant1/1 -> Multiport Switch/1
  neg. edge/1 -> Multiport Switch/3
  pos. edge/1 -> Multiport Switch/2
  In/1 -> Memory/1, NEGATIVE Edge/1(IN), POSITIVE Edge/1(IN)
  Memory/1 -> NEGATIVE Edge/2(IN previous), POSITIVE Edge/2(IN previous)
  POSITIVE Edge/1(OUT) -> Logical Operator1/1
  NEGATIVE Edge/1(OUT) -> Logical Operator1/2
  Logical Operator1/1 -> Out/1

== system powerlib_extras/Control  Blocks/Monostable ==
  note: Silvano Casoria
      | Power System Simulation Laboratory
      | IREQ, Hydro-Quebc
  note: Monostable
  In : Inport  Port=1  LatchInput=off
  Clock : Clock
      settings: Decimation=10
  Edge Detector : Subsystem  mask(Edge Detector){model=EdgeDetect, ic=ic}
      mask prompts: model "Edge:"; ic "Input at t = -eps:"
      mask help:
      | This block compares its present input to its previous input.
      |
      | If the input  is a logic signal (TRUE (1) or FALSE (0), the output is a one-step boolean signal TRUE  when  the specified edge (Rising, Falling or Either)  is detected.
      |
      | This block can also be used to detect the slope polarity of a continuous signal. For example, if the specified edge is  "Rising", the output is TRUE as long as the slope of the input signal is positive.
      |
      | The input value at time preceeding t=0 is specified by the parameter "Input at t=-eps"
      mask init: same as powerlib_extras/Control  Blocks/Edge Detector
      mask Display: plot(0,0,100,100, X1,Y1,X2,Y2,X3,Y3,X4,Y4);
  Logical Operator1 : Logic
  Logical Operator2 : Logic  Orientation=left  Operator=NOT  Inputs=1
  Memory : Memory  Orientation=left  InheritSampleTime=on
  Relational Operator : RelationalOperator  Operator=>  InputSameDT=on
  Sample & Hold : powerlib_extras/Control  Blocks/Sample & Hold  ic=-1e6
  Sum : Sum  SaturateOnIntegerOverflow=on  InputSameDT=on
  T_monostable : Constant  Value=t_mono - eps
  Out : Outport
  wires:
  Logical Operator1/1 -> Sample & Hold/2
  T_monostable/1 -> Sum/2
  Clock/1 -> Sample & Hold/1, Relational Operator/2
  Sum/1 -> Relational Operator/1
  Sample & Hold/1 -> Sum/1
  Memory/1 -> Logical Operator2/1
  Edge Detector/1(Out) -> Logical Operator1/2
  Logical Operator2/1 -> Logical Operator1/1
  Relational Operator/1 -> Memory/1, Out/1
  In/1 -> Edge Detector/1(In)

== system powerlib_extras/Control  Blocks/On/Off Delay ==
  note: On/Off Delay
  note: Silvano Casoria
      | Power System Simulation Laboratory
      | IREQ, Hydro-Quebc
  IN : Inport  Port=1  LatchInput=off
  Clock : Clock
      settings: Decimation=10
  Constant : Constant
  Constant1 : Constant  Value=delay
  Constant2 : Constant  Value=type_delay
  Data Type Conversion1 : DataTypeConversion  OutDataTypeMode=boolean  SaturateOnIntegerOverflow=on  RndMeth=Zero
  Logical Operator1 : Logic  Operator=OR
  Logical Operator2 : Logic  Operator=NOT  Inputs=1
  OFF Delay : Subsystem  TreatAsAtomicUnit=on
  ON Delay : Subsystem  TreatAsAtomicUnit=on
  Relational Operator1 : RelationalOperator  Operator===  InputSameDT=on
  OUT : Outport
  wires:
  Clock/1 -> ON Delay/2(clock), OFF Delay/2(clock)
  IN/1 -> Data Type Conversion1/1
  Constant1/1 -> OFF Delay/3(DELAY), ON Delay/3(DELAY)
  Logical Operator1/1 -> OUT/1
  ON Delay/1(OUT) -> Logical Operator1/1
  OFF Delay/1(OUT) -> Logical Operator1/2
  Logical Operator2/1 -> OFF Delay/Enable
  Constant2/1 -> Relational Operator1/1
  Relational Operator1/1 -> Logical Operator2/1, ON Delay/Enable
  Constant/1 -> Relational Operator1/2
  Data Type Conversion1/1 -> ON Delay/1(IN), OFF Delay/1(IN)
